simulink library "PB_Library_Master"  (R2020b)
settings: Solver=VariableStepAuto  StartTime=0.0  StopTime=10.0  RelTol=1e-3
undefined symbols (not defined in the file): A_M, B_M, E0_M, f_sw, K_M, Q_M, Q_rr, r_c, r_D, R_M, SOC_Init_M, u_ce0, u_D0
libraries: $bdroot x7, Lib_PF_BusLoadDC_TMATS x3, Lib_Dyn_StateSpace_EMTAT x3, TemperatureBlock x1
(part 3 of 3)

== system PB_Library_Master/Boost Converter/DC - DC Converter/Steady State/TemperatureModifiedPerformanceTerm2  ==
  In1 : Inport
  Add5 : Sum  Inputs=+++
  CapacitorResistance : Constant  Value=RC_M
  Constant : Constant  Value=-1/L_M
  Constant1 : Constant  Value=1/C_M
  Constant11 : Constant  Value=-(L_M)
  Constant13 : Constant  Value=0
  Divide1 : Product  Inputs=*/
  "InductorResistance " : Constant  Value=RL_M
  Matrix Concatenate3 : Concatenate  Mode=Multidimensional array
  Matrix Concatenate4 : Concatenate  Mode=Multidimensional array
  Matrix Concatenate5 : Concatenate  Mode=Multidimensional array  ConcatenateDimension=2
  "TModifiedROn " : Subsystem
  Out1 : Outport  VectorParamsAs1DForOutWhenUnconnected=off
  wires:
  Constant/1 -> Matrix Concatenate4/2
  Constant1/1 -> Matrix Concatenate3/1
  CapacitorResistance/1 -> Add5/3
  Matrix Concatenate5/1 -> Out1/1
  In1/1 -> "TModifiedROn "/1(In1)
  "InductorResistance "/1 -> Add5/1
  "TModifiedROn "/1(Out1) -> Add5/2
  Constant13/1 -> Matrix Concatenate4/1
  Matrix Concatenate4/1 -> Matrix Concatenate5/1
  Divide1/1 -> Matrix Concatenate3/2
  Matrix Concatenate3/1 -> Matrix Concatenate5/2
  Add5/1 -> Divide1/1
  Constant11/1 -> Divide1/2

== system PB_Library_Master/Buck Converter/DC - DC Converter/Steady State/TemperatureModifiedPerformanceTerm2  ==
  TAmbient : Inport
  Add5 : Sum  Inputs=+++
  CapacitorResistance : Constant  Value=RC_M
  Constant : Constant  Value=-1/L_M
  Constant1 : Constant  Value=1/C_M
  Constant11 : Constant  Value=-(L_M)
  Constant13 : Constant  Value=0
  Divide1 : Product  Inputs=*/
  "InductorResistance " : Constant  Value=RL_M
  Matrix Concatenate3 : Concatenate  Mode=Multidimensional array
  Matrix Concatenate4 : Concatenate  Mode=Multidimensional array
  Matrix Concatenate5 : Concatenate  Mode=Multidimensional array  ConcatenateDimension=2
  "TModifiedROn " : Subsystem
  Out1 : Outport  VectorParamsAs1DForOutWhenUnconnected=off
  wires:
  Constant/1 -> Matrix Concatenate4/2
  Constant1/1 -> Matrix Concatenate3/1
  CapacitorResistance/1 -> Add5/3
  Matrix Concatenate5/1 -> Out1/1
  TAmbient/1 -> "TModifiedROn "/1(In1)
  "InductorResistance "/1 -> Add5/1
  "TModifiedROn "/1(Out1) -> Add5/2
  Constant13/1 -> Matrix Concatenate4/1
  Matrix Concatenate4/1 -> Matrix Concatenate5/1
  Divide1/1 -> Matrix Concatenate3/2
  Matrix Concatenate3/1 -> Matrix Concatenate5/2
  Add5/1 -> Divide1/1
  Constant11/1 -> Divide1/2

== system PB_Library_Master/Electrothermal_Battery_Model/Battery Core (w// Q)/BatteryCore/BattCapMod  ==
  TAvg : Inport
  "A " : Constant  Value=-9e-05
  Add : Sum  Inputs=+++
  "B " : Constant  Value=0.0071
  Battery Capacity (Ah) : Constant  Value=Q_M
  C : Constant  Value=.868
  Multiply : Product
  Multiply1 : Product
  Multiply2 : Product
  Square : Math  Operator=square  SignedPower=on  SaturateOnIntegerOverflow=on
  BattCapMod : Outport  VectorParamsAs1DForOutWhenUnconnected=off
  wires:
  Multiply2/1 -> BattCapMod/1
  C/1 -> Add/3
  Multiply1/1 -> Add/2
  Add/1 -> Multiply2/2
  "A "/1 -> Multiply/2
  Multiply/1 -> Add/1
  Square/1 -> Multiply/1
  TAvg/1 -> Square/1, Multiply1/1
  Battery Capacity (Ah)/1 -> Multiply2/1
  "B "/1 -> Multiply1/2

== system PB_Library_Master/Electrothermal_Battery_Model/Battery Core (w// Q)/BatteryCore/BattResIMod  ==
  TAvg : Inport
  "A " : Constant  Value=8e-05
  Add : Sum  Inputs=+++
  "B " : Constant  Value=0.0071
  C : Constant  Value=1.1424
  Internal Resistance (Ohm) : Constant  Value=R_M
  Multiply : Product
  Multiply1 : Product
  Multiply2 : Product
  Square : Math  Operator=square  SignedPower=on  SaturateOnIntegerOverflow=on
  BattCapMod : Outport  VectorParamsAs1DForOutWhenUnconnected=off
  wires:
  Multiply2/1 -> BattCapMod/1
  C/1 -> Add/3
  Multiply1/1 -> Add/2
  Add/1 -> Multiply2/2
  "A "/1 -> Multiply/2
  Multiply/1 -> Add/1
  Square/1 -> Multiply/1
  TAvg/1 -> Square/1, Multiply1/1
  Internal Resistance (Ohm)/1 -> Multiply2/1
  "B "/1 -> Multiply1/2

== system PB_Library_Master/Boost Converter/DC - DC Converter/Steady State/TemperatureModifiedPerformanceTerm1 /TModifiedROn  ==
  In1 : Inport
  Add4 : Sum
  Constant10 : Constant  Value=50
  Constant9 : Constant  Value=25
  Divide : Product  Inputs=*/
  Multiply : Product
  "OnResistance " : Constant  Value=Ron_M
  Out1 : Outport  VectorParamsAs1DForOutWhenUnconnected=off
  wires:
  In1/1 -> Add4/1
  Constant10/1 -> Divide/2
  Add4/1 -> Divide/1
  Constant9/1 -> Add4/2
  Divide/1 -> Multiply/2
  Multiply/1 -> Out1/1
  "OnResistance "/1 -> Multiply/1

== system PB_Library_Master/Boost Converter/DC - DC Converter/Steady State/TemperatureModifiedPerformanceTerm2 /TModifiedROn  ==
  In1 : Inport
  Add4 : Sum
  Constant10 : Constant  Value=50
  Constant9 : Constant  Value=25
  Divide : Product  Inputs=*/
  Multiply : Product
  "OnResistance " : Constant  Value=Ron_M
  Out1 : Outport  VectorParamsAs1DForOutWhenUnconnected=off
  wires:
  In1/1 -> Add4/1
  Constant10/1 -> Divide/2
  Add4/1 -> Divide/1
  Constant9/1 -> Add4/2
  Divide/1 -> Multiply/2
  Multiply/1 -> Out1/1
  "OnResistance "/1 -> Multiply/1

== system PB_Library_Master/Buck Converter/DC - DC Converter/Steady State/TemperatureModifiedPerformanceTerm2 /TModifiedROn  ==
  In1 : Inport
  Add4 : Sum
  Constant10 : Constant  Value=50
  Constant9 : Constant  Value=25
  Divide : Product  Inputs=*/
  Multiply : Product
  "OnResistance " : Constant  Value=Ron_M
  Out1 : Outport  VectorParamsAs1DForOutWhenUnconnected=off
  wires:
  In1/1 -> Add4/1
  Constant10/1 -> Divide/2
  Add4/1 -> Divide/1
  Constant9/1 -> Add4/2
  Divide/1 -> Multiply/2
  Multiply/1 -> Out1/1
  "OnResistance "/1 -> Multiply/1

== matlab function PB_Library_Master/Boost Converter/DC - DC Converter/MATLAB Function ==
  data: A1 input; y output; dt input
function y  = switchLogic(A1, dt)    %A1 state martix, dt time step    

StableFlag=all(abs(1+dt*eig(A1))<=1);    %Forward Euler Stability requirement

if StableFlag==1
    y=1;    %runs dynamic model
    
else
    y=0;    %runs steady state model
    
end

end

== matlab function PB_Library_Master/Buck Converter/DC - DC Converter/MATLAB Function ==
  data: A1 input; y output; dt input
function y  = switchLogic(A1, dt)    %A1 state martix, dt time step    

StableFlag=all(abs(1+dt*eig(A1))<=1);    %Forward Euler Stability requirement

if StableFlag==1
    y=1;    %runs dynamic model
    
else
    y=0;    %runs steady state model
    
end

end
